simulink model "GolfSwing3D_SimscapePhysicalInterfaceSwitching"  (R2024b)
settings: Solver=VariableStepAuto  StartTime=0.0  StopTime=StopTime  MaxStep=0.001  RelTol=1e-3
model workspace: external: MAT-File 3DModelInputs.mat (data not in the file)
undefined symbols (not defined in the file): GripStrength, KillswitchFinalValue, KillswitchInitialValue, KillswitchStepTime, LeftLowerArmLength, PlaneTilt, RightLowerArmLength, UpperTorsoLength, X, Y, Z
libraries: nesl_utility x363, sm_lib x137, matrix_library x11, fl_lib x8, simulink x1
(part 7 of 13)

== system GolfSwing3D_SimscapePhysicalInterfaceSwitching/Left Forearm/Left Forearm ==
  Cylindrical Solid1 : sm_lib/Body Elements/Cylindrical Solid  CylinderRadius=1.75  CylinderRadiusUnits=in  CylinderLength=0.5*LeftLowerArmLength  CylinderLengthUnits=in  ExportEntireGeometry=off  InertiaType=CalculateFromGeometry  BasedOnType=Mass  Density=1000  DensityUnits=kg/m^3  Mass=2.5  MassUnits=lbm  CenterOfMass=[0 0 0]  CenterOfMassUnits=m  MomentsOfInertia=[1 1 1]  MomentsOfInertiaUnits=kg*m^2  ProductsOfInertia=[0 0 0]  ProductsOfInertiaUnits=kg*m^2  GraphicType=FromGeometry  MarkerShape=Sphere  MarkerSize=10  GraphicVisPropType=SimpleVisualProperties  GraphicDiffuseColor=[1.0 0.8 0.4]  GraphicOpacity=1.0  GraphicSpecularColor=[0.5 0.5 0.5 1.0]  GraphicAmbientColor=[0.15 0.15 0.15 1.0]  GraphicEmissiveColor=[0.0 0.0 0.0 1.0]  GraphicShininess=75  DoExposeReferenceFrame=off  SerializedFrames=<Frames><Frame><Id>Frame1</Id><Value><Name>Top of Left Forearm</Name><Origin><Source>GeometricFeature</Source><FeatureName>top curve</FeatureName></Origin><PrimaryAxis><DefinedDirection>-X</DefinedDirection><Source>ReferenceFrame</Source><SourceDirection>+Z</SourceDirection><FeatureName></FeatureName></PrimaryAxis><SecondaryAxis><DefinedDirection>+Y</DefinedDirection><Source>ReferenceFrame</Source><SourceDirection>+X</SourceDirection><FeatureName></FeatureName></SecondaryAxis></Value></Frame><Frame><Id>Frame2</Id><Value><Name>Middle of Left Forearm</Name><Origin><Source>GeometricFeature</Source><FeatureName>bottom curve</FeatureName></Origin><PrimaryAxis><DefinedDirection>+Z</DefinedDirection><Source>ReferenceFrame</Source><SourceDirection>+Z</SourceDirection><FeatureName></FeatureName></PrimaryAxis><SecondaryAxis><DefinedDirection>+X</DefinedDirection><Source>ReferenceFrame</Source><SourceDirection>+X</SourceDirection><FeatureName></FeatureName></SecondaryAxis></Value></Frame></Frames>
  Cylindrical Solid2 : sm_lib/Body Elements/Cylindrical Solid  CylinderRadius=1.75  CylinderRadiusUnits=in  CylinderLength=0.5*LeftLowerArmLength  CylinderLengthUnits=in  ExportEntireGeometry=off  InertiaType=CalculateFromGeometry  BasedOnType=Mass  Density=1000  DensityUnits=kg/m^3  Mass=2.5  MassUnits=lbm  CenterOfMass=[0 0 0]  CenterOfMassUnits=m  MomentsOfInertia=[1 1 1]  MomentsOfInertiaUnits=kg*m^2  ProductsOfInertia=[0 0 0]  ProductsOfInertiaUnits=kg*m^2  GraphicType=FromGeometry  MarkerShape=Sphere  MarkerSize=10  GraphicVisPropType=SimpleVisualProperties  GraphicDiffuseColor=[1.0 0.8 0.4]  GraphicOpacity=1.0  GraphicSpecularColor=[0.5 0.5 0.5 1.0]  GraphicAmbientColor=[0.15 0.15 0.15 1.0]  GraphicEmissiveColor=[0.0 0.0 0.0 1.0]  GraphicShininess=75  DoExposeReferenceFrame=off  SerializedFrames=<Frames><Frame><Id>Frame1</Id><Value><Name>Middle of Left Forearm</Name><Origin><Source>GeometricFeature</Source><FeatureName>top curve</FeatureName></Origin><PrimaryAxis><DefinedDirection>-Z</DefinedDirection><Source>ReferenceFrame</Source><SourceDirection>+Z</SourceDirection><FeatureName></FeatureName></PrimaryAxis><SecondaryAxis><DefinedDirection>+X</DefinedDirection><Source>ReferenceFrame</Source><SourceDirection>+X</SourceDirection><FeatureName></FeatureName></SecondaryAxis></Value></Frame><Frame><Id>Frame2</Id><Value><Name>Left Wrist</Name><Origin><Source>GeometricFeature</Source><FeatureName>bottom curve</FeatureName></Origin><PrimaryAxis><DefinedDirection>+Z</DefinedDirection><Source>ReferenceFrame</Source><SourceDirection>+Z</SourceDirection><FeatureName></FeatureName></PrimaryAxis><SecondaryAxis><DefinedDirection>+Y</DefinedDirection><Source>ReferenceFrame</Source><SourceDirection>+Y</SourceDirection><FeatureName></FeatureName></SecondaryAxis></Value></Frame></Frames>
  LF Kinematically Driven : Subsystem  Commented=on
  LF Kinetically Driven : Subsystem
  Rigid Transform : sm_lib/Frames and Transforms/Rigid Transform  RotationMethod=RotationSequence  FollAlignAxisA=+X  BaseAlignAxisA=+Y  FollAlignAxisB=+Y  BaseAlignAxisB=+Z  RotationStandardAxis=+Z  RotationAngle=0  RotationAngleUnits=deg  RotationArbitraryAxis=[0 0 1]  RotationSequenceAxes=FollowerAxes  RotationSequence=XZY  RotationSequenceAngles=[90 180 180]  RotationSequenceAnglesUnits=deg  RotationMatrix=[1 0 0;0 1 0;0 0 1]  Quaternion=[1 0 0 0]  TranslationMethod=None  TranslationCartesianOffset=[0 0 0]  TranslationCartesianOffsetUnits=m  TranslationStandardAxis=+Z  TranslationStandardOffset=0  TranslationStandardOffsetUnits=m  TranslationROffset=0  TranslationROffsetUnits=m  TranslationThetaOffset=0  TranslationThetaOffsetUnits=deg  TranslationZOffset=0  TranslationZOffsetUnits=m
  Rigid Transform2 : sm_lib/Frames and Transforms/Rigid Transform  RotationMethod=RotationSequence  FollAlignAxisA=+X  BaseAlignAxisA=+Y  FollAlignAxisB=+Y  BaseAlignAxisB=+Z  RotationStandardAxis=+Z  RotationAngle=0.0  RotationAngleUnits=deg  RotationArbitraryAxis=[0 0 1]  RotationSequenceAxes=BaseAxes  RotationSequence=XYZ  RotationSequenceAngles=[180 0 90]  RotationSequenceAnglesUnits=deg  RotationMatrix=[1 0 0; 0 1 0; 0 0 1]  Quaternion=[1 0 0 0]  TranslationMethod=None  TranslationCartesianOffset=[0 0 0]  TranslationCartesianOffsetUnits=m  TranslationStandardAxis=+Z  TranslationStandardOffset=0  TranslationStandardOffsetUnits=m  TranslationROffset=0  TranslationROffsetUnits=m  TranslationThetaOffset=0  TranslationThetaOffsetUnits=deg  TranslationZOffset=0  TranslationZOffsetUnits=m
  Top of Left Forearm : PMIOPort  Side=Left
  Left Wrist : PMIOPort  Port=2  Side=Right
  connections:
  Cylindrical Solid2/RConn1 -- Rigid Transform/LConn1
  Cylindrical Solid1/LConn1 -- Top of Left Forearm/RConn1
  Cylindrical Solid1/RConn1 -- Rigid Transform2/LConn1
  Rigid Transform/RConn1 -- Left Wrist/RConn1
  LF Kinematically Driven/RConn1 -- Cylindrical Solid2/LConn1 -- LF Kinetically Driven/RConn1
  LF Kinematically Driven/LConn1 -- Rigid Transform2/RConn1 -- LF Kinetically Driven/LConn1

== system GolfSwing3D_SimscapePhysicalInterfaceSwitching/Left Forearm/Left Forearm MOF ==
  LEAngularImpulseonForearm : Integrator
  LElbowonLForearmMOFGlobal : matrix_library/Cross Product
  LElbowonLForearmMOFLocal : Product  Multiplication=Matrix(*)
  LFCOM : sm_lib/Body Elements/Inertia Sensor  SensorExtent=BodyGroup  SpanWeldJoints=off  ExcludeGroundedBodies=off  MeasurementFrame=World  SenseMass=off  SenseCenterOfMass=on  SenseInertiaMatrix=off  SenseCenteredInertiaMatrix=off  SensePrincipalInertiaMatrix=off  SenseRotationMatrix=off  GraphicType=None  PrincipalInertiaFrameSize=20  GraphicVisPropType=SimpleVisualProperties  GraphicDiffuseColor=[0.5 0.5 0.5]  GraphicOpacity=1  GraphicSpecularColor=[0.5 0.5 0.5 1.0]  GraphicAmbientColor=[0.15 0.15 0.15 1.0]  GraphicEmissiveColor=[0.0 0.0 0.0 1.0]  GraphicShininess=75
  LWristonLForearmMOFGlobal : matrix_library/Cross Product
  LWristonLForearmMOFLocal : Product  Multiplication=Matrix(*)
  Left Forearm COM : nesl_utility/PS-Simulink Converter  PhysicalDomain=network_engine_domain  SubClassName=ps_output  LeftPortType=input  RightPortType=output  PseudoPeriodic=off  Frequencies=[]  VectorFormat=1-D array  Unit=inherit  AffineConversion=off
  R Vector Elbow Force on Left Forearm : Sum  Inputs=-+
  R Vector Wrist Force on Left Forearm : Sum  Inputs=-+
  RotationTransformLeftWrist : nesl_utility/PS-Simulink Converter  PhysicalDomain=network_engine_domain  SubClassName=ps_output  LeftPortType=input  RightPortType=output  PseudoPeriodic=off  Frequencies=[]  VectorFormat=1-D array  Unit=inherit  AffineConversion=off
  SumofMomentsLEonLForearm : Sum
  SumofMomentsLForearmLocal : Product  Multiplication=Matrix(*)
  SumofMomentsLeftForearmGlobal : Sum  Inputs=++++
  Transform Sensor : sm_lib/Frames and Transforms/Transform Sensor  MeasurementFrame=World  RotationSequence=XYX  SenseAngle=off  SenseAxis=off  SenseQ=off  SenseR=on  SenseRotationSequence=off  SenseOmegaX=off  SenseOmegaY=off  SenseOmegaZ=off  SenseOmega=off  SenseQDot=off  SenseRDot=off  SenseRotationSequenceDot=off  SenseAlphaX=off  SenseAlphaY=off  SenseAlphaZ=off  SenseAlpha=off  SenseQDDot=off  SenseRDDot=off  SenseX=off  SenseY=off  SenseZ=off  SenseXYZ=off  SenseRad=off  SenseAzim=off  SenseDist=off  SenseInc=off  SenseXDot=off  SenseYDot=off  SenseZDot=off  SenseXYZDot=off  SenseRadDot=off  SenseAzimDot=off  SenseDistDot=off  SenseIncDot=off  SenseXDDot=off  SenseYDDot=off  SenseZDDot=off  SenseXYZDDot=off  SenseRadDDot=off  SenseAzimDDot=off  SenseDistDDot=off  SenseIncDDot=off
  World Frame : sm_lib/Frames and Transforms/World Frame
  Left Forearm : PMIOPort  Side=Left
  wires:
  Left Forearm COM/1 -> R Vector Elbow Force on Left Forearm/1, R Vector Wrist Force on Left Forearm/1  "LeftForearmCOM"
  [LEGlobalPosition] -> R Vector Elbow Force on Left Forearm/2
  [LWGlobalPosition] -> R Vector Wrist Force on Left Forearm/2
  R Vector Elbow Force on Left Forearm/1 -> LElbowonLForearmMOFGlobal/1
  [LArmonLForearmFGlobalOut] -> LElbowonLForearmMOFGlobal/2
  R Vector Wrist Force on Left Forearm/1 -> LWristonLForearmMOFGlobal/1
  [LHonLWTGlobalOut] -> SumofMomentsLeftForearmGlobal/4
  [LHonLWFGlobalOut] -> LWristonLForearmMOFGlobal/2
  SumofMomentsLeftForearmGlobal/1 -> SumofMomentsLForearmLocal/2  "SumofMomentsLeftForearmGlobal"
  LWristonLForearmMOFGlobal/1 -> LWristonLForearmMOFLocal/2, SumofMomentsLeftForearmGlobal/2  "LWristonLForearmMOFGlobal"
  RotationTransformLeftWrist/1 -> SumofMomentsLForearmLocal/1, LWristonLForearmMOFLocal/1, LElbowonLForearmMOFLocal/1
  LElbowonLForearmMOFGlobal/1 -> SumofMomentsLEonLForearm/2, LElbowonLForearmMOFLocal/2, SumofMomentsLeftForearmGlobal/1  "LElbowonLForearmMOFGlobal"
  SumofMomentsLEonLForearm/1 -> LEAngularImpulseonForearm/1  "SumofMomentsLEonLForearm"
  [LArmonLForearmTGlobalOut] -> SumofMomentsLeftForearmGlobal/3, SumofMomentsLEonLForearm/1
  connections:
  LFCOM/LConn1 -- Transform Sensor/LConn1 -- Left Forearm/RConn1
  LFCOM/RConn1 -- Left Forearm COM/LConn1
  Transform Sensor/RConn1 -- World Frame/RConn1
  RotationTransformLeftWrist/LConn1 -- Transform Sensor/RConn2

== system GolfSwing3D_SimscapePhysicalInterfaceSwitching/Left Scapula Joint/LScap Kinematically Driven ==
  Kinematically Driven LScap : sm_lib/Joints/Universal Joint  JointMode=Normal  CompositeWrenchDir=FollowerOnBase  CompositeWrenchFrame=BaseFrame  SenseConstraintForce=off  SenseConstraintTorque=off  SenseTotalForce=on  SenseTotalTorque=on  RxPositionTargetSpecify=off  RxPositionTargetPriority=Low  RxPositionTargetValue=LScapStartPositionX  RxPositionTargetValueUnits=deg  RxVelocityTargetSpecify=off  RxVelocityTargetPriority=Low  RxVelocityTargetValue=LScapStartVelocityX  RxVelocityTargetValueUnits=deg/s  RxEquilibriumPosition=0  RxEquilibriumPositionUnits=deg  RxSpringStiffness=0  RxSpringStiffnessUnits=N*m/deg  RxDampingCoefficient=0  RxDampingCoefficientUnits=N*m/(deg/s)  RxLowerLimitSpecify=off  RxLowerLimitBound=-30  RxLowerLimitBoundUnits=deg  RxLowerLimitStiffness=200  RxLowerLimitStiffnessUnits=N*m/deg  RxLowerLimitDamping=10  RxLowerLimitDampingUnits=N*m/(deg/s)  RxLowerLimitTransitionRegionWidth=0.1  RxLowerLimitTransitionRegionWidthUnits=deg  RxUpperLimitSpecify=off  RxUpperLimitBound=30  RxUpperLimitBoundUnits=deg  RxUpperLimitStiffness=200  RxUpperLimitStiffnessUnits=N*m/deg  RxUpperLimitDamping=10  RxUpperLimitDampingUnits=N*m/(deg/s)  RxUpperLimitTransitionRegionWidth=0.1  RxUpperLimitTransitionRegionWidthUnits=deg  RxTorqueActuationMode=ComputedTorque  RxMotionActuationMode=InputMotion  RxSensePosition=on  RxSenseVelocity=on  RxSenseAcceleration=off  RxSenseTorqueForce=on  RxSenseLowerLimitTorqueForce=off  RxSenseUpperLimitTorqueForce=off  RyPositionTargetSpecify=off  RyPositionTargetPriority=Low  RyPositionTargetValue=LScapStartPositionY  RyPositionTargetValueUnits=deg  RyVelocityTargetSpecify=off  RyVelocityTargetPriority=Low  RyVelocityTargetValue=LScapStartVelocityY  RyVelocityTargetValueUnits=deg/s  RyEquilibriumPosition=0  RyEquilibriumPositionUnits=deg  RySpringStiffness=0  RySpringStiffnessUnits=N*m/deg  RyDampingCoefficient=0  RyDampingCoefficientUnits=N*m/(deg/s)  RyLowerLimitSpecify=off  RyLowerLimitBound=-30  RyLowerLimitBoundUnits=deg  RyLowerLimitStiffness=200  RyLowerLimitStiffnessUnits=N*m/deg  RyLowerLimitDamping=10  RyLowerLimitDampingUnits=N*m/(deg/s)  RyLowerLimitTransitionRegionWidth=0.1  RyLowerLimitTransitionRegionWidthUnits=deg  RyUpperLimitSpecify=off  RyUpperLimitBound=30  RyUpperLimitBoundUnits=deg  RyUpperLimitStiffness=200  RyUpperLimitStiffnessUnits=N*m/deg  RyUpperLimitDamping=10  RyUpperLimitDampingUnits=N*m/(deg/s)  RyUpperLimitTransitionRegionWidth=0.1  RyUpperLimitTransitionRegionWidthUnits=deg  RyTorqueActuationMode=ComputedTorque  RyMotionActuationMode=InputMotion  RySensePosition=on  RySenseVelocity=on  RySenseAcceleration=off  RySenseTorqueForce=on  RySenseLowerLimitTorqueForce=off  RySenseUpperLimitTorqueForce=off
  LScapForceLocal : nesl_utility/PS-Simulink Converter  PhysicalDomain=network_engine_domain  SubClassName=ps_output  LeftPortType=input  RightPortType=output  PseudoPeriodic=off  Frequencies=[]  VectorFormat=1-D array  Unit=inherit  AffineConversion=off
  LScapPositionX : nesl_utility/PS-Simulink Converter  PhysicalDomain=network_engine_domain  SubClassName=ps_output  LeftPortType=input  RightPortType=output  PseudoPeriodic=off  Frequencies=[]  VectorFormat=1-D array  Unit=deg  AffineConversion=off
  LScapPositionY : nesl_utility/PS-Simulink Converter  PhysicalDomain=network_engine_domain  SubClassName=ps_output  LeftPortType=input  RightPortType=output  PseudoPeriodic=off  Frequencies=[]  VectorFormat=1-D array  Unit=deg  AffineConversion=off
  LScapTorqueLocal : nesl_utility/PS-Simulink Converter  PhysicalDomain=network_engine_domain  SubClassName=ps_output  LeftPortType=input  RightPortType=output  PseudoPeriodic=off  Frequencies=[]  VectorFormat=1-D array  Unit=inherit  AffineConversion=off
  LScapTorqueXInput : nesl_utility/PS-Simulink Converter  PhysicalDomain=network_engine_domain  SubClassName=ps_output  LeftPortType=input  RightPortType=output  PseudoPeriodic=off  Frequencies=[]  VectorFormat=1-D array  Unit=inherit  AffineConversion=off
  LScapTorqueYInput : nesl_utility/PS-Simulink Converter  PhysicalDomain=network_engine_domain  SubClassName=ps_output  LeftPortType=input  RightPortType=output  PseudoPeriodic=off  Frequencies=[]  VectorFormat=1-D array  Unit=inherit  AffineConversion=off
  LScapVelocityX : nesl_utility/PS-Simulink Converter  PhysicalDomain=network_engine_domain  SubClassName=ps_output  LeftPortType=input  RightPortType=output  PseudoPeriodic=off  Frequencies=[]  VectorFormat=1-D array  Unit=deg/s  AffineConversion=off
  LScapVelocityY : nesl_utility/PS-Simulink Converter  PhysicalDomain=network_engine_domain  SubClassName=ps_output  LeftPortType=input  RightPortType=output  PseudoPeriodic=off  Frequencies=[]  VectorFormat=1-D array  Unit=deg/s  AffineConversion=off
  Simulink-PS Converter12 : nesl_utility/Simulink-PS Converter  PhysicalDomain=network_engine_domain  SubClassName=ps_input  LeftPortType=input  RightPortType=output  PseudoPeriodic=off  Frequencies=[]  NoiseDistribution=none  NoiseParameters=[]  Unit=deg  AffineConversion=off  FilteringAndDerivatives=provide  SimscapeFilterOrder=1  InputFilterTimeConstant=0.001  UdotUserProvided=2
  Simulink-PS Converter13 : nesl_utility/Simulink-PS Converter  PhysicalDomain=network_engine_domain  SubClassName=ps_input  LeftPortType=input  RightPortType=output  PseudoPeriodic=off  Frequencies=[]  NoiseDistribution=none  NoiseParameters=[]  Unit=deg  AffineConversion=off  FilteringAndDerivatives=provide  SimscapeFilterOrder=1  InputFilterTimeConstant=0.001  UdotUserProvided=2
  Conn1 : PMIOPort  Side=Left
  Conn2 : PMIOPort  Port=2  Side=Right
  tag scope: LScapPositionX=global, LScapPositionY=global, LScapVelocityX=global, LScapVelocityY=global
  wires:
  [FcnOutLScapVelocityX] -> Simulink-PS Converter12/2
  LScapPositionY/1 -> [LScapPositionY]  "LScapPositionY"
  LScapPositionX/1 -> [LScapPositionX]  "LScapPositionX"
  [FcnOutLScapPositionX] -> Simulink-PS Converter12/1
  [FcnOutLScapVelocityY] -> Simulink-PS Converter13/2
  [FcnOutLScapAccelerationY] -> Simulink-PS Converter13/3
  [FcnOutLScapPositionY] -> Simulink-PS Converter13/1
  [FcnOutLScapAccelerationX] -> Simulink-PS Converter12/3
  LScapVelocityY/1 -> [LScapVelocityY]  "LScapVelocityY"
  LScapVelocityX/1 -> [LScapVelocityX]  "LScapVelocityX"
  LScapTorqueLocal/1 -> ?  "LScapTorqueLocal"
  LScapTorqueXInput/1 -> ?  "LScapTorqueXInput"
  LScapTorqueYInput/1 -> ?  "LScapTorqueYInput"
  connections:
  Kinematically Driven LScap/LConn3 -- Simulink-PS Converter13/RConn1
  LScapTorqueLocal/LConn1 -- Kinematically Driven LScap/RConn9
  Kinematically Driven LScap/RConn1 -- Conn2/RConn1
  LScapVelocityY/LConn1 -- Kinematically Driven LScap/RConn6
  Simulink-PS Converter12/RConn1 -- Kinematically Driven LScap/LConn2
  LScapPositionX/LConn1 -- Kinematically Driven LScap/RConn2
  LScapVelocityX/LConn1 -- Kinematically Driven LScap/RConn3
  LScapForceLocal/LConn1 -- Kinematically Driven LScap/RConn8
  LScapPositionY/LConn1 -- Kinematically Driven LScap/RConn5
  Kinematically Driven LScap/LConn1 -- Conn1/RConn1
  LScapTorqueYInput/LConn1 -- Kinematically Driven LScap/RConn7
  LScapTorqueXInput/LConn1 -- Kinematically Driven LScap/RConn4

== system GolfSwing3D_SimscapePhysicalInterfaceSwitching/Left Scapula Joint/LScap Kinetically Driven ==
  Kinetically Driven LScap : sm_lib/Joints/Universal Joint  JointMode=Normal  CompositeWrenchDir=FollowerOnBase  CompositeWrenchFrame=BaseFrame  SenseConstraintForce=off  SenseConstraintTorque=off  SenseTotalForce=on  SenseTotalTorque=on  RxPositionTargetSpecify=on  RxPositionTargetPriority=Low  RxPositionTargetValue=LScapStartPositionX  RxPositionTargetValueUnits=deg  RxVelocityTargetSpecify=on  RxVelocityTargetPriority=Low  RxVelocityTargetValue=LScapStartVelocityX  RxVelocityTargetValueUnits=deg/s  RxEquilibriumPosition=0  RxEquilibriumPositionUnits=deg  RxSpringStiffness=0  RxSpringStiffnessUnits=N*m/deg  RxDampingCoefficient=0  RxDampingCoefficientUnits=N*m/(deg/s)  RxLowerLimitSpecify=off  RxLowerLimitBound=-30  RxLowerLimitBoundUnits=deg  RxLowerLimitStiffness=200  RxLowerLimitStiffnessUnits=N*m/deg  RxLowerLimitDamping=10  RxLowerLimitDampingUnits=N*m/(deg/s)  RxLowerLimitTransitionRegionWidth=0.1  RxLowerLimitTransitionRegionWidthUnits=deg  RxUpperLimitSpecify=off  RxUpperLimitBound=30  RxUpperLimitBoundUnits=deg  RxUpperLimitStiffness=200  RxUpperLimitStiffnessUnits=N*m/deg  RxUpperLimitDamping=10  RxUpperLimitDampingUnits=N*m/(deg/s)  RxUpperLimitTransitionRegionWidth=0.1  RxUpperLimitTransitionRegionWidthUnits=deg  RxTorqueActuationMode=InputTorque  RxMotionActuationMode=ComputedMotion  RxSensePosition=on  RxSenseVelocity=on  RxSenseAcceleration=off  RxSenseTorqueForce=on  RxSenseLowerLimitTorqueForce=off  RxSenseUpperLimitTorqueForce=off  RyPositionTargetSpecify=on  RyPositionTargetPriority=Low  RyPositionTargetValue=LScapStartPositionY  RyPositionTargetValueUnits=deg  RyVelocityTargetSpecify=on  RyVelocityTargetPriority=Low  RyVelocityTargetValue=LScapStartVelocityY  RyVelocityTargetValueUnits=deg/s  RyEquilibriumPosition=0  RyEquilibriumPositionUnits=deg  RySpringStiffness=0  RySpringStiffnessUnits=N*m/deg  RyDampingCoefficient=0  RyDampingCoefficientUnits=N*m/(deg/s)  RyLowerLimitSpecify=off  RyLowerLimitBound=-30  RyLowerLimitBoundUnits=deg  RyLowerLimitStiffness=200  RyLowerLimitStiffnessUnits=N*m/deg  RyLowerLimitDamping=10  RyLowerLimitDampingUnits=N*m/(deg/s)  RyLowerLimitTransitionRegionWidth=0.1  RyLowerLimitTransitionRegionWidthUnits=deg  RyUpperLimitSpecify=off  RyUpperLimitBound=30  RyUpperLimitBoundUnits=deg  RyUpperLimitStiffness=200  RyUpperLimitStiffnessUnits=N*m/deg  RyUpperLimitDamping=10  RyUpperLimitDampingUnits=N*m/(deg/s)  RyUpperLimitTransitionRegionWidth=0.1  RyUpperLimitTransitionRegionWidthUnits=deg  RyTorqueActuationMode=InputTorque  RyMotionActuationMode=ComputedMotion  RySensePosition=on  RySenseVelocity=on  RySenseAcceleration=off  RySenseTorqueForce=on  RySenseLowerLimitTorqueForce=off  RySenseUpperLimitTorqueForce=off
  LScapForceLocal : nesl_utility/PS-Simulink Converter  PhysicalDomain=network_engine_domain  SubClassName=ps_output  LeftPortType=input  RightPortType=output  PseudoPeriodic=off  Frequencies=[]  VectorFormat=1-D array  Unit=inherit  AffineConversion=off
  LScapPositionX : nesl_utility/PS-Simulink Converter  PhysicalDomain=network_engine_domain  SubClassName=ps_output  LeftPortType=input  RightPortType=output  PseudoPeriodic=off  Frequencies=[]  VectorFormat=1-D array  Unit=deg  AffineConversion=off
  LScapPositionY : nesl_utility/PS-Simulink Converter  PhysicalDomain=network_engine_domain  SubClassName=ps_output  LeftPortType=input  RightPortType=output  PseudoPeriodic=off  Frequencies=[]  VectorFormat=1-D array  Unit=deg  AffineConversion=off
  LScapTorqueLocal : nesl_utility/PS-Simulink Converter  PhysicalDomain=network_engine_domain  SubClassName=ps_output  LeftPortType=input  RightPortType=output  PseudoPeriodic=off  Frequencies=[]  VectorFormat=1-D array  Unit=inherit  AffineConversion=off
  LScapTorqueXInput : nesl_utility/PS-Simulink Converter  PhysicalDomain=network_engine_domain  SubClassName=ps_output  LeftPortType=input  RightPortType=output  PseudoPeriodic=off  Frequencies=[]  VectorFormat=1-D array  Unit=inherit  AffineConversion=off
  LScapTorqueYInput : nesl_utility/PS-Simulink Converter  PhysicalDomain=network_engine_domain  SubClassName=ps_output  LeftPortType=input  RightPortType=output  PseudoPeriodic=off  Frequencies=[]  VectorFormat=1-D array  Unit=inherit  AffineConversion=off
  LScapVelocityX : nesl_utility/PS-Simulink Converter  PhysicalDomain=network_engine_domain  SubClassName=ps_output  LeftPortType=input  RightPortType=output  PseudoPeriodic=off  Frequencies=[]  VectorFormat=1-D array  Unit=deg/s  AffineConversion=off
  LScapVelocityY : nesl_utility/PS-Simulink Converter  PhysicalDomain=network_engine_domain  SubClassName=ps_output  LeftPortType=input  RightPortType=output  PseudoPeriodic=off  Frequencies=[]  VectorFormat=1-D array  Unit=deg/s  AffineConversion=off
  LeftScapTorque : nesl_utility/Simulink-PS Converter  PhysicalDomain=network_engine_domain  SubClassName=ps_input  LeftPortType=input  RightPortType=output  PseudoPeriodic=off  Frequencies=[]  NoiseDistribution=none  NoiseParameters=[]  Unit=N*m  AffineConversion=off  FilteringAndDerivatives=provide  SimscapeFilterOrder=1  InputFilterTimeConstant=0.001  UdotUserProvided=0
  LeftScapTorqueY : nesl_utility/Simulink-PS Converter  PhysicalDomain=network_engine_domain  SubClassName=ps_input  LeftPortType=input  RightPortType=output  PseudoPeriodic=off  Frequencies=[]  NoiseDistribution=none  NoiseParameters=[]  Unit=N*m  AffineConversion=off  FilteringAndDerivatives=provide  SimscapeFilterOrder=1  InputFilterTimeConstant=0.001  UdotUserProvided=0
  Conn1 : PMIOPort  Side=Left
  Conn2 : PMIOPort  Port=2  Side=Right
  tag scope: LScapPositionX=global, LScapPositionY=global, LScapVelocityX=global, LScapVelocityY=global
  wires:
  LScapVelocityX/1 -> [LScapVelocityX]  "LScapVelocityX"
  [FcnOutLScapTorqueY] -> LeftScapTorqueY/1
  LScapVelocityY/1 -> [LScapVelocityY]  "LScapVelocityY"
  LScapPositionY/1 -> [LScapPositionY]  "LScapPositionY"
  LScapPositionX/1 -> [LScapPositionX]  "LScapPositionX"
  [FcnOutLScapTorqueX] -> LeftScapTorque/1
  LScapTorqueLocal/1 -> ?  "LScapTorqueLocal"
  LScapTorqueXInput/1 -> ?  "LScapTorqueXInput"
  LScapTorqueYInput/1 -> ?  "LScapTorqueYInput"
  connections:
  Kinetically Driven LScap/RConn2 -- LScapPositionX/LConn1
  Kinetically Driven LScap/RConn3 -- LScapVelocityX/LConn1
  Kinetically Driven LScap/RConn6 -- LScapVelocityY/LConn1
  Conn1/RConn1 -- Kinetically Driven LScap/LConn1
  LeftScapTorque/RConn1 -- Kinetically Driven LScap/LConn2
  Kinetically Driven LScap/RConn5 -- LScapPositionY/LConn1
  LScapForceLocal/LConn1 -- Kinetically Driven LScap/RConn8
  LeftScapTorqueY/RConn1 -- Kinetically Driven LScap/LConn3
  Conn2/RConn1 -- Kinetically Driven LScap/RConn1
  LScapTorqueYInput/LConn1 -- Kinetically Driven LScap/RConn7
  LScapTorqueXInput/LConn1 -- Kinetically Driven LScap/RConn4
  LScapTorqueLocal/LConn1 -- Kinetically Driven LScap/RConn9

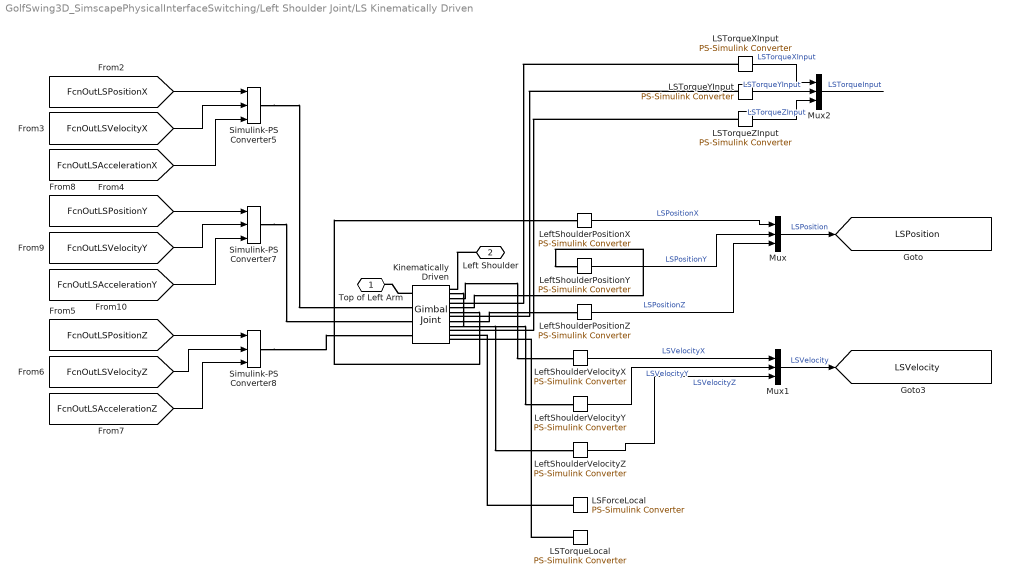
== system GolfSwing3D_SimscapePhysicalInterfaceSwitching/Left Shoulder Joint/LS Kinematically Driven ==
  Kinematically Driven : sm_lib/Joints/Gimbal Joint  JointMode=Normal  CompositeWrenchDir=BaseOnFollower  CompositeWrenchFrame=FollowerFrame  SenseConstraintForce=off  SenseConstraintTorque=off  SenseTotalForce=on  SenseTotalTorque=on  RxPositionTargetSpecify=off  RxPositionTargetPriority=Low  RxPositionTargetValue=LSStartPositionX  RxPositionTargetValueUnits=deg  RxVelocityTargetSpecify=off  RxVelocityTargetPriority=Low  RxVelocityTargetValue=LSStartVelocityX  RxVelocityTargetValueUnits=deg/s  RxEquilibriumPosition=120  RxEquilibriumPositionUnits=deg  RxSpringStiffness=0  RxSpringStiffnessUnits=N*m/deg  RxDampingCoefficient=0  RxDampingCoefficientUnits=N*m/(deg/s)  RxLowerLimitSpecify=off  RxLowerLimitBound=-80  RxLowerLimitBoundUnits=deg  RxLowerLimitStiffness=100  RxLowerLimitStiffnessUnits=N*m/deg  RxLowerLimitDamping=10  RxLowerLimitDampingUnits=N*m/(deg/s)  RxLowerLimitTransitionRegionWidth=0.1  RxLowerLimitTransitionRegionWidthUnits=deg  RxUpperLimitSpecify=off  RxUpperLimitBound=80  RxUpperLimitBoundUnits=deg  RxUpperLimitStiffness=100  RxUpperLimitStiffnessUnits=N*m/deg  RxUpperLimitDamping=10  RxUpperLimitDampingUnits=N*m/(deg/s)  RxUpperLimitTransitionRegionWidth=0.1  RxUpperLimitTransitionRegionWidthUnits=deg  RxTorqueActuationMode=ComputedTorque  RxMotionActuationMode=InputMotion  RxSensePosition=on  RxSenseVelocity=on  RxSenseAcceleration=off  RxSenseTorqueForce=on  RxSenseLowerLimitTorqueForce=off  RxSenseUpperLimitTorqueForce=off  RyPositionTargetSpecify=off  RyPositionTargetPriority=Low  RyPositionTargetValue=LSStartPositionY  RyPositionTargetValueUnits=deg  RyVelocityTargetSpecify=off  RyVelocityTargetPriority=Low  RyVelocityTargetValue=LSStartVelocityY  RyVelocityTargetValueUnits=deg/s  RyEquilibriumPosition=0  RyEquilibriumPositionUnits=deg  RySpringStiffness=0  RySpringStiffnessUnits=N*m/deg  RyDampingCoefficient=0  RyDampingCoefficientUnits=N*m/(deg/s)  RyLowerLimitSpecify=off  RyLowerLimitBound=-80  RyLowerLimitBoundUnits=deg  RyLowerLimitStiffness=100  RyLowerLimitStiffnessUnits=N*m/deg  RyLowerLimitDamping=10  RyLowerLimitDampingUnits=N*m/(deg/s)  RyLowerLimitTransitionRegionWidth=0.1  RyLowerLimitTransitionRegionWidthUnits=deg  RyUpperLimitSpecify=off  RyUpperLimitBound=80  RyUpperLimitBoundUnits=deg  RyUpperLimitStiffness=100  RyUpperLimitStiffnessUnits=N*m/deg  RyUpperLimitDamping=10  RyUpperLimitDampingUnits=N*m/(deg/s)  RyUpperLimitTransitionRegionWidth=0.1  RyUpperLimitTransitionRegionWidthUnits=deg  RyTorqueActuationMode=ComputedTorque  RyMotionActuationMode=InputMotion  RySensePosition=on  RySenseVelocity=on  RySenseAcceleration=off  RySenseTorqueForce=on  RySenseLowerLimitTorqueForce=off  RySenseUpperLimitTorqueForce=off  RzPositionTargetSpecify=off  RzPositionTargetPriority=Low  RzPositionTargetValue=LSStartPositionZ  RzPositionTargetValueUnits=deg  RzVelocityTargetSpecify=off  RzVelocityTargetPriority=Low  RzVelocityTargetValue=LSStartVelocityZ  RzVelocityTargetValueUnits=deg/s  RzEquilibriumPosition=0  RzEquilibriumPositionUnits=deg  RzSpringStiffness=0  RzSpringStiffnessUnits=N*m/deg  RzDampingCoefficient=0  RzDampingCoefficientUnits=N*m/(deg/s)  RzLowerLimitSpecify=off  RzLowerLimitBound=-180  RzLowerLimitBoundUnits=deg  RzLowerLimitStiffness=100  RzLowerLimitStiffnessUnits=N*m/deg  RzLowerLimitDamping=10  RzLowerLimitDampingUnits=N*m/(deg/s)  RzLowerLimitTransitionRegionWidth=0.1  RzLowerLimitTransitionRegionWidthUnits=deg  RzUpperLimitSpecify=off  RzUpperLimitBound=-95  RzUpperLimitBoundUnits=deg  RzUpperLimitStiffness=100  RzUpperLimitStiffnessUnits=N*m/deg  RzUpperLimitDamping=10  RzUpperLimitDampingUnits=N*m/(deg/s)  RzUpperLimitTransitionRegionWidth=0.1  RzUpperLimitTransitionRegionWidthUnits=deg  RzTorqueActuationMode=ComputedTorque  RzMotionActuationMode=InputMotion  RzSensePosition=on  RzSenseVelocity=on  RzSenseAcceleration=off  RzSenseTorqueForce=on  RzSenseLowerLimitTorqueForce=off  RzSenseUpperLimitTorqueForce=off
  LSForceLocal : nesl_utility/PS-Simulink Converter  PhysicalDomain=network_engine_domain  SubClassName=ps_output  LeftPortType=input  RightPortType=output  PseudoPeriodic=off  Frequencies=[]  VectorFormat=1-D array  Unit=inherit  AffineConversion=off
  LSTorqueLocal : nesl_utility/PS-Simulink Converter  PhysicalDomain=network_engine_domain  SubClassName=ps_output  LeftPortType=input  RightPortType=output  PseudoPeriodic=off  Frequencies=[]  VectorFormat=1-D array  Unit=inherit  AffineConversion=off
  LSTorqueXInput : nesl_utility/PS-Simulink Converter  PhysicalDomain=network_engine_domain  SubClassName=ps_output  LeftPortType=input  RightPortType=output  PseudoPeriodic=off  Frequencies=[]  VectorFormat=1-D array  Unit=inherit  AffineConversion=off
  LSTorqueYInput : nesl_utility/PS-Simulink Converter  PhysicalDomain=network_engine_domain  SubClassName=ps_output  LeftPortType=input  RightPortType=output  PseudoPeriodic=off  Frequencies=[]  VectorFormat=1-D array  Unit=inherit  AffineConversion=off
  LSTorqueZInput : nesl_utility/PS-Simulink Converter  PhysicalDomain=network_engine_domain  SubClassName=ps_output  LeftPortType=input  RightPortType=output  PseudoPeriodic=off  Frequencies=[]  VectorFormat=1-D array  Unit=inherit  AffineConversion=off
  LeftShoulderPositionX : nesl_utility/PS-Simulink Converter  PhysicalDomain=network_engine_domain  SubClassName=ps_output  LeftPortType=input  RightPortType=output  PseudoPeriodic=off  Frequencies=[]  VectorFormat=1-D array  Unit=deg  AffineConversion=off
  LeftShoulderPositionY : nesl_utility/PS-Simulink Converter  PhysicalDomain=network_engine_domain  SubClassName=ps_output  LeftPortType=input  RightPortType=output  PseudoPeriodic=off  Frequencies=[]  VectorFormat=1-D array  Unit=deg  AffineConversion=off
  LeftShoulderPositionZ : nesl_utility/PS-Simulink Converter  PhysicalDomain=network_engine_domain  SubClassName=ps_output  LeftPortType=input  RightPortType=output  PseudoPeriodic=off  Frequencies=[]  VectorFormat=1-D array  Unit=deg  AffineConversion=off
  LeftShoulderVelocityX : nesl_utility/PS-Simulink Converter  PhysicalDomain=network_engine_domain  SubClassName=ps_output  LeftPortType=input  RightPortType=output  PseudoPeriodic=off  Frequencies=[]  VectorFormat=1-D array  Unit=deg/s  AffineConversion=off
  LeftShoulderVelocityY : nesl_utility/PS-Simulink Converter  PhysicalDomain=network_engine_domain  SubClassName=ps_output  LeftPortType=input  RightPortType=output  PseudoPeriodic=off  Frequencies=[]  VectorFormat=1-D array  Unit=deg/s  AffineConversion=off
  LeftShoulderVelocityZ : nesl_utility/PS-Simulink Converter  PhysicalDomain=network_engine_domain  SubClassName=ps_output  LeftPortType=input  RightPortType=output  PseudoPeriodic=off  Frequencies=[]  VectorFormat=1-D array  Unit=deg/s  AffineConversion=off
  Mux : Mux  Inputs=3
  Mux1 : Mux  Inputs=3
  Mux2 : Mux  Inputs=3
  Simulink-PS Converter5 : nesl_utility/Simulink-PS Converter  PhysicalDomain=network_engine_domain  SubClassName=ps_input  LeftPortType=input  RightPortType=output  PseudoPeriodic=off  Frequencies=[]  NoiseDistribution=none  NoiseParameters=[]  Unit=deg  AffineConversion=off  FilteringAndDerivatives=provide  SimscapeFilterOrder=1  InputFilterTimeConstant=0.001  UdotUserProvided=2
  Simulink-PS Converter7 : nesl_utility/Simulink-PS Converter  PhysicalDomain=network_engine_domain  SubClassName=ps_input  LeftPortType=input  RightPortType=output  PseudoPeriodic=off  Frequencies=[]  NoiseDistribution=none  NoiseParameters=[]  Unit=deg  AffineConversion=off  FilteringAndDerivatives=provide  SimscapeFilterOrder=1  InputFilterTimeConstant=0.001  UdotUserProvided=2
  Simulink-PS Converter8 : nesl_utility/Simulink-PS Converter  PhysicalDomain=network_engine_domain  SubClassName=ps_input  LeftPortType=input  RightPortType=output  PseudoPeriodic=off  Frequencies=[]  NoiseDistribution=none  NoiseParameters=[]  Unit=deg  AffineConversion=off  FilteringAndDerivatives=provide  SimscapeFilterOrder=1  InputFilterTimeConstant=0.001  UdotUserProvided=2
  Top of Left Arm : PMIOPort  Side=Left
  Left Shoulder : PMIOPort  Port=2  Side=Right
  tag scope: LSPosition=global, LSVelocity=global
  wires:
  [FcnOutLSPositionX] -> Simulink-PS Converter5/1
  [FcnOutLSPositionZ] -> Simulink-PS Converter8/1
  [FcnOutLSPositionY] -> Simulink-PS Converter7/1
  [FcnOutLSAccelerationZ] -> Simulink-PS Converter8/3
  [FcnOutLSAccelerationX] -> Simulink-PS Converter5/3
  [FcnOutLSAccelerationY] -> Simulink-PS Converter7/3
  [FcnOutLSVelocityY] -> Simulink-PS Converter7/2
  [FcnOutLSVelocityX] -> Simulink-PS Converter5/2
  [FcnOutLSVelocityZ] -> Simulink-PS Converter8/2
  LeftShoulderPositionY/1 -> Mux/2  "LSPositionY"
  LeftShoulderVelocityY/1 -> Mux1/2  "LSVelocityY"
  LeftShoulderPositionZ/1 -> Mux/3  "LSPositionZ"
  LeftShoulderVelocityX/1 -> Mux1/1  "LSVelocityX"
  LeftShoulderPositionX/1 -> Mux/1  "LSPositionX"
  LeftShoulderVelocityZ/1 -> Mux1/3  "LSVelocityZ"
  Mux/1 -> [LSPosition]  "LSPosition"
  Mux1/1 -> [LSVelocity]  "LSVelocity"
  LSTorqueXInput/1 -> Mux2/1  "LSTorqueXInput"
  LSTorqueYInput/1 -> Mux2/2  "LSTorqueYInput"
  LSTorqueZInput/1 -> Mux2/3  "LSTorqueZInput"
  Mux2/1 -> ?  "LSTorqueInput"
  connections:
  Kinematically Driven/LConn1 -- Top of Left Arm/RConn1
  Simulink-PS Converter5/RConn1 -- Kinematically Driven/LConn2
  Simulink-PS Converter7/RConn1 -- Kinematically Driven/LConn3
  Simulink-PS Converter8/RConn1 -- Kinematically Driven/LConn4
  Left Shoulder/RConn1 -- Kinematically Driven/RConn1
  Kinematically Driven/RConn2 -- LeftShoulderPositionX/LConn1
  Kinematically Driven/RConn5 -- LeftShoulderPositionY/LConn1
  Kinematically Driven/RConn8 -- LeftShoulderPositionZ/LConn1
  Kinematically Driven/RConn3 -- LeftShoulderVelocityX/LConn1
  Kinematically Driven/RConn6 -- LeftShoulderVelocityY/LConn1
  Kinematically Driven/RConn9 -- LeftShoulderVelocityZ/LConn1
  LSForceLocal/LConn1 -- Kinematically Driven/RConn11
  LSTorqueLocal/LConn1 -- Kinematically Driven/RConn12
  LSTorqueXInput/LConn1 -- Kinematically Driven/RConn4
  LSTorqueYInput/LConn1 -- Kinematically Driven/RConn7
  LSTorqueZInput/LConn1 -- Kinematically Driven/RConn10

== system GolfSwing3D_SimscapePhysicalInterfaceSwitching/Left Shoulder Joint/LS Kinetically Driven ==
  Kinetically Driven : sm_lib/Joints/Gimbal Joint  JointMode=Normal  CompositeWrenchDir=BaseOnFollower  CompositeWrenchFrame=FollowerFrame  SenseConstraintForce=off  SenseConstraintTorque=off  SenseTotalForce=on  SenseTotalTorque=on  RxPositionTargetSpecify=on  RxPositionTargetPriority=Low  RxPositionTargetValue=LSStartPositionX  RxPositionTargetValueUnits=deg  RxVelocityTargetSpecify=on  RxVelocityTargetPriority=Low  RxVelocityTargetValue=LSStartVelocityX  RxVelocityTargetValueUnits=deg/s  RxEquilibriumPosition=120  RxEquilibriumPositionUnits=deg  RxSpringStiffness=0  RxSpringStiffnessUnits=N*m/deg  RxDampingCoefficient=0  RxDampingCoefficientUnits=N*m/(deg/s)  RxLowerLimitSpecify=off  RxLowerLimitBound=-80  RxLowerLimitBoundUnits=deg  RxLowerLimitStiffness=100  RxLowerLimitStiffnessUnits=N*m/deg  RxLowerLimitDamping=10  RxLowerLimitDampingUnits=N*m/(deg/s)  RxLowerLimitTransitionRegionWidth=0.1  RxLowerLimitTransitionRegionWidthUnits=deg  RxUpperLimitSpecify=off  RxUpperLimitBound=80  RxUpperLimitBoundUnits=deg  RxUpperLimitStiffness=100  RxUpperLimitStiffnessUnits=N*m/deg  RxUpperLimitDamping=10  RxUpperLimitDampingUnits=N*m/(deg/s)  RxUpperLimitTransitionRegionWidth=0.1  RxUpperLimitTransitionRegionWidthUnits=deg  RxTorqueActuationMode=InputTorque  RxMotionActuationMode=ComputedMotion  RxSensePosition=on  RxSenseVelocity=on  RxSenseAcceleration=off  RxSenseTorqueForce=on  RxSenseLowerLimitTorqueForce=off  RxSenseUpperLimitTorqueForce=off  RyPositionTargetSpecify=on  RyPositionTargetPriority=Low  RyPositionTargetValue=LSStartPositionY  RyPositionTargetValueUnits=deg  RyVelocityTargetSpecify=on  RyVelocityTargetPriority=Low  RyVelocityTargetValue=LSStartVelocityY  RyVelocityTargetValueUnits=deg/s  RyEquilibriumPosition=0  RyEquilibriumPositionUnits=deg  RySpringStiffness=0  RySpringStiffnessUnits=N*m/deg  RyDampingCoefficient=0  RyDampingCoefficientUnits=N*m/(deg/s)  RyLowerLimitSpecify=off  RyLowerLimitBound=-80  RyLowerLimitBoundUnits=deg  RyLowerLimitStiffness=100  RyLowerLimitStiffnessUnits=N*m/deg  RyLowerLimitDamping=10  RyLowerLimitDampingUnits=N*m/(deg/s)  RyLowerLimitTransitionRegionWidth=0.1  RyLowerLimitTransitionRegionWidthUnits=deg  RyUpperLimitSpecify=off  RyUpperLimitBound=80  RyUpperLimitBoundUnits=deg  RyUpperLimitStiffness=100  RyUpperLimitStiffnessUnits=N*m/deg  RyUpperLimitDamping=10  RyUpperLimitDampingUnits=N*m/(deg/s)  RyUpperLimitTransitionRegionWidth=0.1  RyUpperLimitTransitionRegionWidthUnits=deg  RyTorqueActuationMode=InputTorque  RyMotionActuationMode=ComputedMotion  RySensePosition=on  RySenseVelocity=on  RySenseAcceleration=off  RySenseTorqueForce=on  RySenseLowerLimitTorqueForce=off  RySenseUpperLimitTorqueForce=off  RzPositionTargetSpecify=on  RzPositionTargetPriority=Low  RzPositionTargetValue=LSStartPositionZ  RzPositionTargetValueUnits=deg  RzVelocityTargetSpecify=on  RzVelocityTargetPriority=Low  RzVelocityTargetValue=LSStartVelocityZ  RzVelocityTargetValueUnits=deg/s  RzEquilibriumPosition=0  RzEquilibriumPositionUnits=deg  RzSpringStiffness=0  RzSpringStiffnessUnits=N*m/deg  RzDampingCoefficient=0  RzDampingCoefficientUnits=N*m/(deg/s)  RzLowerLimitSpecify=off  RzLowerLimitBound=-180  RzLowerLimitBoundUnits=deg  RzLowerLimitStiffness=100  RzLowerLimitStiffnessUnits=N*m/deg  RzLowerLimitDamping=10  RzLowerLimitDampingUnits=N*m/(deg/s)  RzLowerLimitTransitionRegionWidth=0.1  RzLowerLimitTransitionRegionWidthUnits=deg  RzUpperLimitSpecify=off  RzUpperLimitBound=-95  RzUpperLimitBoundUnits=deg  RzUpperLimitStiffness=100  RzUpperLimitStiffnessUnits=N*m/deg  RzUpperLimitDamping=10  RzUpperLimitDampingUnits=N*m/(deg/s)  RzUpperLimitTransitionRegionWidth=0.1  RzUpperLimitTransitionRegionWidthUnits=deg  RzTorqueActuationMode=InputTorque  RzMotionActuationMode=ComputedMotion  RzSensePosition=on  RzSenseVelocity=on  RzSenseAcceleration=off  RzSenseTorqueForce=on  RzSenseLowerLimitTorqueForce=off  RzSenseUpperLimitTorqueForce=off
  LSForceLocal : nesl_utility/PS-Simulink Converter  PhysicalDomain=network_engine_domain  SubClassName=ps_output  LeftPortType=input  RightPortType=output  PseudoPeriodic=off  Frequencies=[]  VectorFormat=1-D array  Unit=inherit  AffineConversion=off
  LSTorqueLocal : nesl_utility/PS-Simulink Converter  PhysicalDomain=network_engine_domain  SubClassName=ps_output  LeftPortType=input  RightPortType=output  PseudoPeriodic=off  Frequencies=[]  VectorFormat=1-D array  Unit=inherit  AffineConversion=off
  LSTorqueXInput : nesl_utility/PS-Simulink Converter  PhysicalDomain=network_engine_domain  SubClassName=ps_output  LeftPortType=input  RightPortType=output  PseudoPeriodic=off  Frequencies=[]  VectorFormat=1-D array  Unit=inherit  AffineConversion=off
  LSTorqueYInput : nesl_utility/PS-Simulink Converter  PhysicalDomain=network_engine_domain  SubClassName=ps_output  LeftPortType=input  RightPortType=output  PseudoPeriodic=off  Frequencies=[]  VectorFormat=1-D array  Unit=inherit  AffineConversion=off
  LSTorqueZInput : nesl_utility/PS-Simulink Converter  PhysicalDomain=network_engine_domain  SubClassName=ps_output  LeftPortType=input  RightPortType=output  PseudoPeriodic=off  Frequencies=[]  VectorFormat=1-D array  Unit=inherit  AffineConversion=off
  Left Shoulder Torque : nesl_utility/Simulink-PS Converter  PhysicalDomain=network_engine_domain  SubClassName=ps_input  LeftPortType=input  RightPortType=output  PseudoPeriodic=off  Frequencies=[]  NoiseDistribution=none  NoiseParameters=[]  Unit=N*m  AffineConversion=off  FilteringAndDerivatives=provide  SimscapeFilterOrder=1  InputFilterTimeConstant=0.001  UdotUserProvided=0
  LeftShoulderPositionX : nesl_utility/PS-Simulink Converter  PhysicalDomain=network_engine_domain  SubClassName=ps_output  LeftPortType=input  RightPortType=output  PseudoPeriodic=off  Frequencies=[]  VectorFormat=1-D array  Unit=deg  AffineConversion=off
  LeftShoulderPositionY : nesl_utility/PS-Simulink Converter  PhysicalDomain=network_engine_domain  SubClassName=ps_output  LeftPortType=input  RightPortType=output  PseudoPeriodic=off  Frequencies=[]  VectorFormat=1-D array  Unit=deg  AffineConversion=off
  LeftShoulderPositionZ : nesl_utility/PS-Simulink Converter  PhysicalDomain=network_engine_domain  SubClassName=ps_output  LeftPortType=input  RightPortType=output  PseudoPeriodic=off  Frequencies=[]  VectorFormat=1-D array  Unit=deg  AffineConversion=off
  LeftShoulderVelocityX : nesl_utility/PS-Simulink Converter  PhysicalDomain=network_engine_domain  SubClassName=ps_output  LeftPortType=input  RightPortType=output  PseudoPeriodic=off  Frequencies=[]  VectorFormat=1-D array  Unit=deg/s  AffineConversion=off
  LeftShoulderVelocityY : nesl_utility/PS-Simulink Converter  PhysicalDomain=network_engine_domain  SubClassName=ps_output  LeftPortType=input  RightPortType=output  PseudoPeriodic=off  Frequencies=[]  VectorFormat=1-D array  Unit=deg/s  AffineConversion=off
  LeftShoulderVelocityZ : nesl_utility/PS-Simulink Converter  PhysicalDomain=network_engine_domain  SubClassName=ps_output  LeftPortType=input  RightPortType=output  PseudoPeriodic=off  Frequencies=[]  VectorFormat=1-D array  Unit=deg/s  AffineConversion=off
  Mux : Mux  Inputs=3
  Mux1 : Mux  Inputs=3
  Mux2 : Mux  Inputs=3
  Simulink-PS Converter2 : nesl_utility/Simulink-PS Converter  PhysicalDomain=network_engine_domain  SubClassName=ps_input  LeftPortType=input  RightPortType=output  PseudoPeriodic=off  Frequencies=[]  NoiseDistribution=none  NoiseParameters=[]  Unit=1  AffineConversion=off  FilteringAndDerivatives=provide  SimscapeFilterOrder=1  InputFilterTimeConstant=0.001  UdotUserProvided=0
  Simulink-PS Converter6 : nesl_utility/Simulink-PS Converter  PhysicalDomain=network_engine_domain  SubClassName=ps_input  LeftPortType=input  RightPortType=output  PseudoPeriodic=off  Frequencies=[]  NoiseDistribution=none  NoiseParameters=[]  Unit=1  AffineConversion=off  FilteringAndDerivatives=provide  SimscapeFilterOrder=1  InputFilterTimeConstant=0.001  UdotUserProvided=0
  Top of Left Arm : PMIOPort  Side=Left
  Left Shoulder : PMIOPort  Port=2  Side=Right
  LSForceLocalOut : PMIOPort  Port=3  Side=Right
  LSTorqueLocalOut : PMIOPort  Port=4  Side=Right
  tag scope: LSPosition=global, LSVelocity=global
  wires:
  LeftShoulderVelocityZ/1 -> Mux1/3  "LSVelocityZ"
  [FcnOutLSTorqueZ] -> Left Shoulder Torque/1
  LeftShoulderPositionY/1 -> Mux/2  "LSPositionY"
  [FcnOutLSTorqueY] -> Simulink-PS Converter6/1
  LeftShoulderPositionZ/1 -> Mux/3  "LSPositionZ"
  LeftShoulderVelocityY/1 -> Mux1/2  "LSVelocityY"
  LeftShoulderPositionX/1 -> Mux/1  "LSPositionX"
  LeftShoulderVelocityX/1 -> Mux1/1  "LSVelocityX"
  [FcnOutLSTorqueX] -> Simulink-PS Converter2/1
  Mux/1 -> [LSPosition]  "LSPosition"
  Mux1/1 -> [LSVelocity]  "LSVelocity"
  LSTorqueXInput/1 -> Mux2/1  "LSTorqueXInput"
  LSTorqueYInput/1 -> Mux2/2  "LSTorqueYInput"
  LSTorqueZInput/1 -> Mux2/3  "LSTorqueZInput"
  Mux2/1 -> ?  "LSTorqueInput"
  connections:
  Kinetically Driven/RConn3 -- LeftShoulderVelocityX/LConn1
  Simulink-PS Converter6/RConn1 -- Kinetically Driven/LConn3
  LSForceLocalOut/RConn1 -- LSForceLocal/LConn1 -- Kinetically Driven/RConn11
  LeftShoulderPositionX/LConn1 -- Kinetically Driven/RConn2
  Simulink-PS Converter2/RConn1 -- Kinetically Driven/LConn2
  LeftShoulderPositionZ/LConn1 -- Kinetically Driven/RConn8
  Left Shoulder Torque/RConn1 -- Kinetically Driven/LConn4
  LSTorqueLocalOut/RConn1 -- Kinetically Driven/RConn12 -- LSTorqueLocal/LConn1
  LeftShoulderVelocityY/LConn1 -- Kinetically Driven/RConn6
  LeftShoulderVelocityZ/LConn1 -- Kinetically Driven/RConn9
  Kinetically Driven/RConn5 -- LeftShoulderPositionY/LConn1
  Top of Left Arm/RConn1 -- Kinetically Driven/LConn1
  Left Shoulder/RConn1 -- Kinetically Driven/RConn1
  LSTorqueZInput/LConn1 -- Kinetically Driven/RConn10
  LSTorqueXInput/LConn1 -- Kinetically Driven/RConn4
  LSTorqueYInput/LConn1 -- Kinetically Driven/RConn7

== system GolfSwing3D_SimscapePhysicalInterfaceSwitching/Left Upper Arm/Left Upper Arm MOF ==
  LElbowonLArmMOFLocal : Product  Multiplication=Matrix(*)
  LSAngularImpulseonArm : Integrator
  LShoulderonLArmMOFGlobal : matrix_library/Cross Product
  LShoulderonLArmMOFLocal : Product  Multiplication=Matrix(*)
  LUACOM : sm_lib/Body Elements/Inertia Sensor  SensorExtent=BodyGroup  SpanWeldJoints=off  ExcludeGroundedBodies=off  MeasurementFrame=World  SenseMass=off  SenseCenterOfMass=on  SenseInertiaMatrix=on  SenseCenteredInertiaMatrix=off  SensePrincipalInertiaMatrix=off  SenseRotationMatrix=off  GraphicType=PrincipalInertiaFrame  PrincipalInertiaFrameSize=20  GraphicVisPropType=SimpleVisualProperties  GraphicDiffuseColor=[0.5 0.5 0.5]  GraphicOpacity=1  GraphicSpecularColor=[0.5 0.5 0.5 1.0]  GraphicAmbientColor=[0.15 0.15 0.15 1.0]  GraphicEmissiveColor=[0.0 0.0 0.0 1.0]  GraphicShininess=75
  Left Upper Arm COM : nesl_utility/PS-Simulink Converter  PhysicalDomain=network_engine_domain  SubClassName=ps_output  LeftPortType=input  RightPortType=output  PseudoPeriodic=off  Frequencies=[]  VectorFormat=1-D array  Unit=inherit  AffineConversion=off
  LeftElbowonLArmMOFGlobal : matrix_library/Cross Product
  R Vector Elbow Force on Left Arm : Sum  Inputs=-+
  R Vector Shoulder Force on Left Arm : Sum  Inputs=-+
  Rotation Transform Left Arm : nesl_utility/PS-Simulink Converter  PhysicalDomain=network_engine_domain  SubClassName=ps_output  LeftPortType=input  RightPortType=output  PseudoPeriodic=off  Frequencies=[]  VectorFormat=1-D array  Unit=inherit  AffineConversion=off
  SumofMomentsLArmLocal : Product  Multiplication=Matrix(*)
  SumofMomentsLSonLArm : Sum
  SumofMomentsLeftArmGlobal : Sum  Inputs=++++
  Transform Sensor : sm_lib/Frames and Transforms/Transform Sensor  MeasurementFrame=World  RotationSequence=XYX  SenseAngle=off  SenseAxis=off  SenseQ=off  SenseR=on  SenseRotationSequence=off  SenseOmegaX=off  SenseOmegaY=off  SenseOmegaZ=off  SenseOmega=off  SenseQDot=off  SenseRDot=off  SenseRotationSequenceDot=off  SenseAlphaX=off  SenseAlphaY=off  SenseAlphaZ=off  SenseAlpha=off  SenseQDDot=off  SenseRDDot=off  SenseX=off  SenseY=off  SenseZ=off  SenseXYZ=off  SenseRad=off  SenseAzim=off  SenseDist=off  SenseInc=off  SenseXDot=off  SenseYDot=off  SenseZDot=off  SenseXYZDot=off  SenseRadDot=off  SenseAzimDot=off  SenseDistDot=off  SenseIncDot=off  SenseXDDot=off  SenseYDDot=off  SenseZDDot=off  SenseXYZDDot=off  SenseRadDDot=off  SenseAzimDDot=off  SenseDistDDot=off  SenseIncDDot=off
  World Frame : sm_lib/Frames and Transforms/World Frame
  Left Upper Arm : PMIOPort  Side=Left
  wires:
  Left Upper Arm COM/1 -> R Vector Shoulder Force on Left Arm/1, R Vector Elbow Force on Left Arm/1  "LUpperArmCOM"
  [LEGlobalPosition] -> R Vector Elbow Force on Left Arm/2
  R Vector Elbow Force on Left Arm/1 -> LeftElbowonLArmMOFGlobal/1
  R Vector Shoulder Force on Left Arm/1 -> LShoulderonLArmMOFGlobal/1
  [LSGlobalPosition] -> R Vector Shoulder Force on Left Arm/2
  [LSonLArmFGlobalOut] -> LShoulderonLArmMOFGlobal/2
  [LForearmonLArmFGlobalOut] -> LeftElbowonLArmMOFGlobal/2
  [LForearmonLArmTGlobalOut] -> SumofMomentsLeftArmGlobal/4
  [LSonLArmTGlobalOut] -> SumofMomentsLSonLArm/1, SumofMomentsLeftArmGlobal/3
  Rotation Transform Left Arm/1 -> SumofMomentsLArmLocal/1, LElbowonLArmMOFLocal/1, LShoulderonLArmMOFLocal/1
  LShoulderonLArmMOFGlobal/1 -> SumofMomentsLeftArmGlobal/1, SumofMomentsLSonLArm/2, LShoulderonLArmMOFLocal/2  "LShoulderonLArmMOFGlobal"
  LeftElbowonLArmMOFGlobal/1 -> SumofMomentsLeftArmGlobal/2, LElbowonLArmMOFLocal/2  "LElbowonLArmMOFGlobal"
  SumofMomentsLeftArmGlobal/1 -> SumofMomentsLArmLocal/2  "SumofMomentsLeftArmGlobal"
  SumofMomentsLSonLArm/1 -> LSAngularImpulseonArm/1  "SumofMomentsLSonLArm"
  connections:
  LUACOM/LConn1 -- Transform Sensor/LConn1 -- Left Upper Arm/RConn1
  Left Upper Arm COM/LConn1 -- LUACOM/RConn1
  Transform Sensor/RConn1 -- World Frame/RConn1
  Rotation Transform Left Arm/LConn1 -- Transform Sensor/RConn2
